simulink subsystem "Wiper"  (R2023b)
settings: Solver=VariableStepAuto  StartTime=0.0  StopTime=10.0  RelTol=1e-3
settings Model: Creator=Asus  LastModifiedBy=Asus

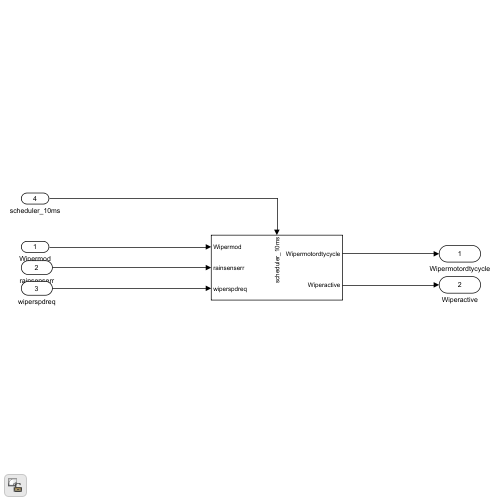
[thumbnail: Simulink's stored preview of the top-level diagram]
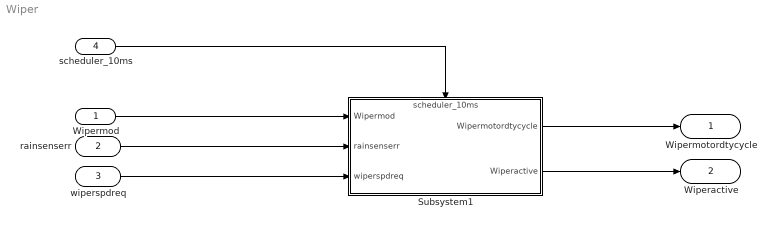
== system Wiper ==
  Wipermod : Inport  OutDataTypeStr=uint8
  rainsenserr : Inport  Port=2  OutDataTypeStr=boolean
  wiperspdreq : Inport  Port=3  OutDataTypeStr=uint8
  scheduler_10ms : Inport  Port=4  OutDataTypeStr=uint8
  Subsystem1 : Subsystem
      settings: PortSchema="{\"entries\":[{\"content\":{\"sides\":[{\"content\":{\"connectorIds\":[\"In1\",\"In2\",\"In3\"]},\"type\":\"ConnectorPlacement.EquallySpacedRectSide\",\"uuid\":\"7af3442d-0cbe-409e-a655-6cb0b5f6116b\"},{\"content\":{\"connectorIds\":[\"Out1\",\"Out2\"],\"side\":\"RIGHT\"},\"type\":\"ConnectorPlacement.EquallySpacedRectSide\",\"uuid\":\"27834f24-1a0f-4e44-91b4-b0b9d5126f86\"},{\"content\":{\"connectorIds\":[\"In4\"],\"side\":\"TOP\"},\"type\":\"ConnectorPlacement.EquallySpacedRectSide\",\"uuid\":\"3a577dad-3d7f-403b-b823-6580cb165d70\"}]},\"type\":\"ConnectorPlacement.EquallySpacedConnector\",\"uuid\":\"6e6197cc-0880-4190-90f2-9f3def51bfa9\"}],\"packageUris\":[\"http://schema.mathworks.com/mf0/Connector/R2020b\"],\"version\":\"1.0\"}"
  Wipermotordtycycle : Outport  OutDataTypeStr=single
  Wiperactive : Outport  Port=2  OutDataTypeStr=boolean
  wires:
  scheduler_10ms/1 -> Subsystem1/4(scheduler_10ms)
  Subsystem1/2(Wiperactive) -> Wiperactive/1
  wiperspdreq/1 -> Subsystem1/3(wiperspdreq)
  Subsystem1/1(Wipermotordtycycle) -> Wipermotordtycycle/1
  rainsenserr/1 -> Subsystem1/2(rainsenserr)
  Wipermod/1 -> Subsystem1/1(Wipermod)

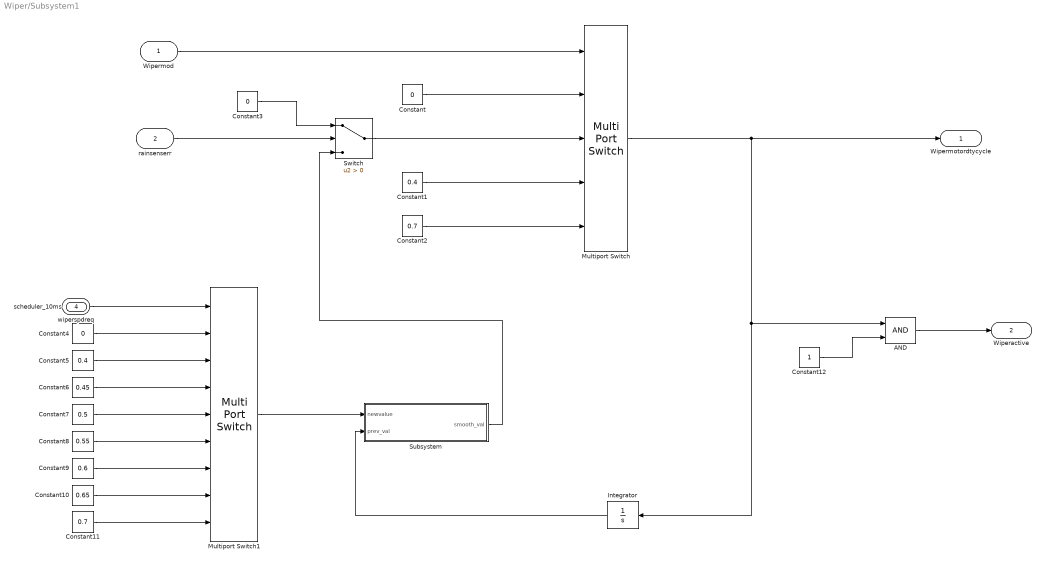
== system Wiper/Subsystem1 ==
  Wipermod : Inport  OutDataTypeStr=uint8
  rainsenserr : Inport  Port=2  OutDataTypeStr=boolean
  wiperspdreq : Inport  Port=3  OutDataTypeStr=uint8
  scheduler_10ms : Inport  Port=4
  AND : Logic  IconShape=distinctive  AllPortsSameDT=off  OutDataTypeStr=boolean
  Constant : Constant  Value=0
  Constant1 : Constant  Value=0.4
  Constant10 : Constant  Value=0.65
  Constant11 : Constant  Value=0.7
  Constant12 : Constant
  Constant2 : Constant  Value=0.7
  Constant3 : Constant  Value=0
  Constant4 : Constant  Value=0
  Constant5 : Constant  Value=0.4
  Constant6 : Constant  Value=0.45
  Constant7 : Constant  Value=0.5
  Constant8 : Constant  Value=0.55
  Constant9 : Constant  Value=0.6
  Integrator : Integrator
  Multiport Switch : MultiPortSwitch  DataPortOrder=Zero-based contiguous  Inputs=4  zeroidx=on  SaturateOnIntegerOverflow=off  InputSameDT=off
  Multiport Switch1 : MultiPortSwitch  DataPortOrder=Zero-based contiguous  Inputs=8  zeroidx=on  SaturateOnIntegerOverflow=off  InputSameDT=off
  Subsystem : Subsystem
  Switch : Switch  Criteria=u2 > Threshold  SaturateOnIntegerOverflow=off  InputSameDT=off
  Wipermotordtycycle : Outport
  Wiperactive : Outport  Port=2
  wires:
  Subsystem/1(smooth_val) -> Switch/3
  Multiport Switch1/1 -> Subsystem/1(newvalue)
  rainsenserr/1 -> Switch/2
  wiperspdreq/1 -> Multiport Switch1/1
  Integrator/1 -> Subsystem/2(prev_val)
  Constant11/1 -> Multiport Switch1/9
  Constant7/1 -> Multiport Switch1/5
  Constant8/1 -> Multiport Switch1/6
  Constant9/1 -> Multiport Switch1/7
  Constant3/1 -> Switch/1
  Constant2/1 -> Multiport Switch/5
  Constant1/1 -> Multiport Switch/4
  Constant4/1 -> Multiport Switch1/2
  Constant6/1 -> Multiport Switch1/4
  Constant/1 -> Multiport Switch/2
  Constant10/1 -> Multiport Switch1/8
  Constant5/1 -> Multiport Switch1/3
  Multiport Switch/1 -> Integrator/1, AND/1, Wipermotordtycycle/1
  Constant12/1 -> AND/2
  AND/1 -> Wiperactive/1
  Wipermod/1 -> Multiport Switch/1
  Switch/1 -> Multiport Switch/3

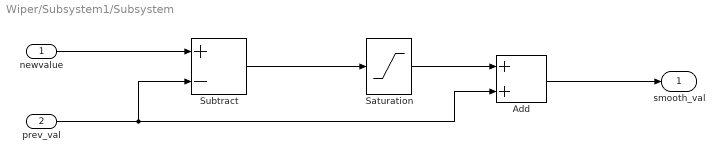
== system Wiper/Subsystem1/Subsystem ==
  newvalue : Inport
  prev_val : Inport  Port=2
  Add : Sum
  Saturation : Saturate  UpperLimit=0.005  LowerLimit=-0.005  ZeroCross=off
  Subtract : Sum  Inputs=+-
  smooth_val : Outport
  wires:
  Add/1 -> smooth_val/1
  prev_val/1 -> Add/2, Subtract/2
  Saturation/1 -> Add/1
  Subtract/1 -> Saturation/1
  newvalue/1 -> Subtract/1
